simulink model "c02_SubAdc"  (R2024a)
settings: Solver=FixedStepDiscrete  StartTime=0.0  StopTime=1  FixedStep=mSim.dTime  MaxStep=Define.sModelSampleTime  RelTol=7.1420e-05
undefined symbols (not defined in the file): C02IGBTS, C02ITLKV, C02MTLKV, C02MTRTS, CnstNr
libraries: Lib_LPF x2
settings Model: Creator=user  LastModifiedBy=admin
settings SolverCC: MaxConsecutiveZCs=10000  ZeroCrossAlgorithm=Adaptive  AlgebraicLoopSolver=TrustRegion
settings DataIOCC: SaveOutput=off  DSMLogging=off  InspectSignalLogs=on  SaveTime=off  SignalLoggingName=logsout_Validator
settings OptimizationCC: BlockReduction=off  DefaultParameterBehavior=Inlined  UseDivisionForNetSlopeComputation=UseDivisionForReciprocalsOfIntegersOnly  GainParamInheritBuiltInType=on  UseFloatMulNetSlope=on  DefaultUnderspecifiedDataType=single  InlineInvariantSignals=on  BitwiseOrLogicalOp=Logical operator  PassReuseOutputArgsAs=Individual arguments  EfficientFloat2IntCast=on  LifeSpan=Inf  OptimizeBlockOrder=speed  DifferentSizesBufferReuse=on  EfficientTunableParamExpr=on
settings DebuggingCC: SignalInfNanChecking=error  SignalRangeChecking=error  ReadBeforeWriteMsg=EnableAllAsError  WriteAfterWriteMsg=EnableAllAsError  WriteAfterReadMsg=EnableAllAsError  AlgebraicLoopMsg=error  ArtificialAlgebraicLoopMsg=error  SaveWithDisabledLinksMsg=error  SaveWithParameterizedLinksMsg=error  BlockPriorityViolationMsg=error  SolverPrmCheckMsg=error  InheritedTsInSrcMsg=error  SingleTaskRateTransMsg=error  TasksWithSamePriorityMsg=error  SigSpecEnsureSampleTimeMsg=error  CheckMatrixSingularityMsg=error  IntegerOverflowMsg=error  ParameterUnderflowMsg=error  ParameterPrecisionLossMsg=error  ParameterTunabilityLossMsg=error  UnderSpecifiedDataTypeMsg=error  UnnecessaryDatatypeConvMsg=warning  VectorMatrixConversionMsg=error  SignalLabelMismatchMsg=error  UnconnectedInputMsg=error  UnconnectedOutputMsg=error  UnconnectedLineMsg=error  SFcnCompatibilityMsg=error  UniqueDataStoreMsg=error  BusObjectLabelMismatch=error  RootOutportRequireBusObject=error  AssertControl=DisableAll  ModelReferenceIOMismatchMessage=error  UnknownTsInhSupMsg=error  ModelReferenceDataLoggingMessage=error  ModelReferenceSymbolNameMessage=none  StateNameClashWarn=warning  StrictBusMsg=ErrorOnBusTreatedAsVector  NonBusSignalsTreatedAsBus=error  SFInvalidInputDataAccessInChartInitDiag=error  SFTransitionOutsideNaturalParentDiag=error  SFUnreachableExecutionPathDiag=error  SFUndirectedBroadcastEventsDiag=error  SFTransitionActionBeforeConditionDiag=error  SFTemporalDelaySmallerThanSampleTimeDiag=error  SFSelfTransitionDiag=error  SFExecutionAtInitializationDiag=error  IntegerSaturationMsg=error  UnitsInconsistencyMsg=none  VariantConditionMismatch=error
settings HardwareCC: ProdBitPerChar=16  ProdBitPerInt=16  ProdBitPerPointer=32  ProdBitPerSizeT=32  ProdBitPerPtrDiffT=32  ProdLargestAtomicInteger=Integer  ProdLargestAtomicFloat=None  ProdWordSize=16  ProdHWDeviceType=Texas Instruments->C2000
settings ModelReferenceCC: EnableRefExpFcnMdlSchedulingChecks=on  ModelReferenceNumInstancesAllowed=Single
settings SFSimCC: SimUseLocalCustomCode=off  CompileTimeRecursionLimit=0  EnableRuntimeRecursion=off  MATLABDynamicMemAlloc=off  CustomCodeUndefinedFunction=UseInterfaceOnly
settings RTWCC: Description=Embedded Coder  SystemTargetFile=ert.tlc  GenCodeOnly=on  TemplateMakefile=ert_default_tmf  GenerateReport=on  RTWUseLocalCustomCode=off  BuildConfiguration=Faster Runs  IncludeHyperlinkInReport=on  LaunchReport=on  GenerateTraceInfo=on  GenerateTraceReport=on  GenerateTraceReportSl=on  GenerateTraceReportSf=on  GenerateWebview=on  GenerateCodeMetricsReport=on  GenerateCodeReplacementReport=on  GPUComputeCapability=3.5  DLArmComputeVersion=19.05
settings CodeAppCC: ForceParamTrailComments=on  IgnoreCustomStorageClasses=off  MATLABFcnDesc=on  MangleLength=4  CustomSymbolStrGlobalVar=GvC02$N$M  CustomSymbolStrType=StrC02$N$M  CustomSymbolStrFcn=$N$M$F  CustomSymbolStrMacro=$N$M  DefineNamingRule=UpperCase  ParamNamingRule=UpperCase  SimulinkBlockComments=off  MATLABSourceComments=on  EnableCustomComments=on  ReqsInCode=on
settings ERTTargetCC: TargetLangStandard=C99 (ISO)  UtilityFuncGeneration=Shared location  MultiwordLength=2048  IncludeMdlTerminateFcn=off  CombineSignalStateStructs=on  SuppressErrorStatus=on  SupportAbsoluteTime=off  SupportNonFinite=off  ParenthesesLevel=Maximum  CastingMode=Standards  GenerateSharedConstants=off  InlinedParameterPlacement=NonHierarchical  ERTSrcFileBannerTemplate=t_code_template.cgt  ERTHdrFileBannerTemplate=t_code_template.cgt  ERTDataSrcFileTemplate=t_code_template.cgt  ERTDataHdrFileTemplate=t_code_template.cgt  ERTCustomFileTemplate=example_file_process.tlc  ERTFilePackagingFormat=CompactWithDataFile  PreserveExpressionOrder=on  SuppressUnreachableDefaultCases=off  EnableSignedLeftShifts=off  EnableSignedRightShifts=off  IndentStyle=Allman  IndentSize=4
settings ConfigComp: CovSaveName=coveragedata  CovMetricSettings=we  CovEnableCumulative=off  CovSaveCumulativeToWorkspaceVar=on  CovSaveSingleToWorkspaceVar=on  CovOutputDir=sldv_output/$ModelName$\sldv_covoutput  PSVerificationMode=BugFinder  PSModelRefIgnoreList=[]  PSEnableModelRefIgnoreList=off  PSModelRefMinMaxVerif=CheckAndConstrain  PSAutoStubLUT=on  DVModelCoverageObjectives=MCDC  DVTestSuiteOptimization=CombinedObjectives (Nonlinear Extended)  DVRebuildModelRepresentation=Always
settings SimscapeCC: SimscapeNormalizeSystem=off

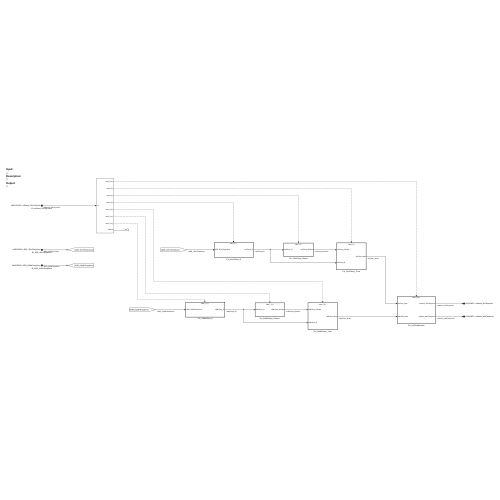
[thumbnail: Simulink's stored preview of the top-level diagram]
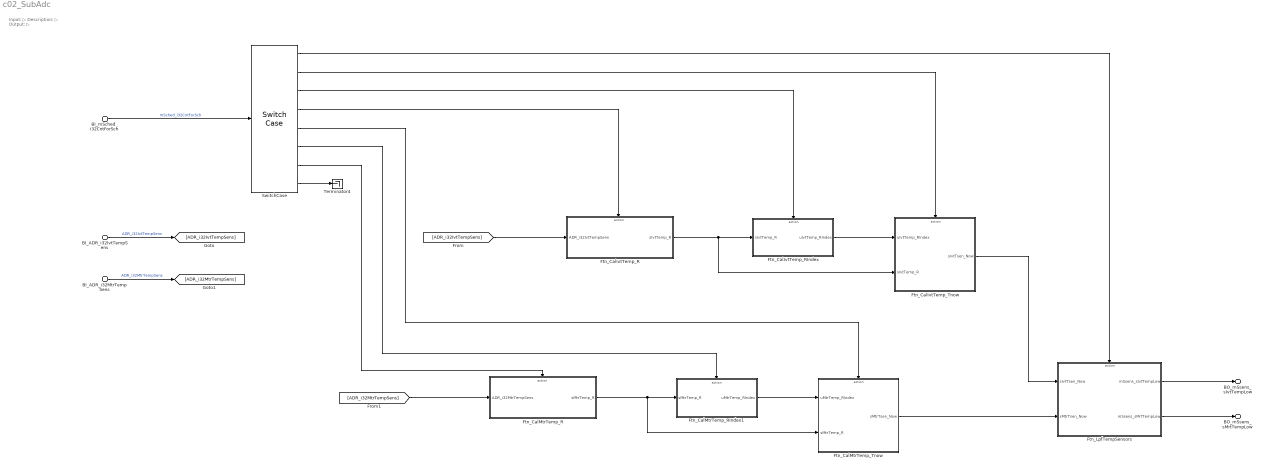
== system c02_SubAdc ==
  note: Input:
      | ▷
      | Description:
      | ▷
      | Output:
      | ▷
  BI_ADR_i32IvtTempSens : Inport  Description=■ 설명: IGBT 온도 센서 ADCV  PortName=bADCREAD  Element=ADR_i32IvtTempSens
  BI_ADR_i32MtrTempSens : Inport  Description=■ 설명: 모터 온도 센서 ADCV  PortName=bADCREAD  Element=ADR_i32MtrTempSens
  BI_mSched_i32CntForSch : Inport  Description=■ 설명: 메인 스케쥴 카운터  Port=2  PortName=bB01SCHED  Element=mSched_i32CntForSch
  Ftn_CalIvtTemp_R : Subsystem
      settings: RTWSystemCode=Nonreusable function  RTWFcnNameOpts=Use subsystem name
  Ftn_CalIvtTemp_RIndex : Subsystem
      settings: RTWSystemCode=Nonreusable function  RTWFcnNameOpts=Use subsystem name
  Ftn_CalIvtTemp_Tnow : Subsystem
      settings: RTWSystemCode=Nonreusable function  RTWFcnNameOpts=Use subsystem name
  Ftn_CalMtrTemp_R : Subsystem
      settings: RTWSystemCode=Nonreusable function  RTWFcnNameOpts=Use subsystem name
  Ftn_CalMtrTemp_RIndex1 : Subsystem
      settings: RTWSystemCode=Nonreusable function  RTWFcnNameOpts=Use subsystem name
  Ftn_CalMtrTemp_Tnow : Subsystem
      settings: RTWSystemCode=Nonreusable function  RTWFcnNameOpts=Use subsystem name
  Ftn_LpfTempSensors : Subsystem
  SwitchCase : SwitchCase  CaseConditions={22, 6,4,2,16,14,12}
  Terminator4 : Terminator
  BO_mSsens_sIvtTempLow : Outport  Description=■ 설명: IGBT 온도  PortName=bC02SADC  Element=mSsens_sIvtTempLow
  BO_mSsens_sMrtTempLow : Outport  Description=■ 설명: 모터 온도  PortName=bC02SADC  Element=mSsens_sMrtTempLow
  wires:
  BI_ADR_i32IvtTempSens/1 -> [ADR_i32IvtTempSens]  "ADR_i32IvtTempSens"
  BI_mSched_i32CntForSch/1 -> SwitchCase/1  "mSched_i32CntForSch"
  Ftn_CalIvtTemp_R/1(sIvtTemp_R) -> Ftn_CalIvtTemp_RIndex/1(sIvtTemp_R), Ftn_CalIvtTemp_Tnow/2(sIvtTemp_R)
  Ftn_CalIvtTemp_RIndex/1(uIvtTemp_RIndex) -> Ftn_CalIvtTemp_Tnow/1(uIvtTemp_RIndex)
  SwitchCase/2 -> Ftn_CalIvtTemp_Tnow/Action
  SwitchCase/3 -> Ftn_CalIvtTemp_RIndex/Action
  SwitchCase/4 -> Ftn_CalIvtTemp_R/Action
  [ADR_i32IvtTempSens] -> Ftn_CalIvtTemp_R/1(ADR_i32IvtTempSens)
  Ftn_CalIvtTemp_Tnow/1(sIvtTsen_Now) -> Ftn_LpfTempSensors/1(sIvtTsen_Now)
  BI_ADR_i32MtrTempSens/1 -> [ADR_i32MtrTempSens]  "ADR_i32MtrTempSens"
  SwitchCase/8 -> Terminator4/1
  SwitchCase/1 -> Ftn_LpfTempSensors/Action
  Ftn_LpfTempSensors/1(mSsens_sIvtTempLow) -> BO_mSsens_sIvtTempLow/1
  Ftn_LpfTempSensors/2(mSsens_sMrtTempLow) -> BO_mSsens_sMrtTempLow/1
  Ftn_CalMtrTemp_Tnow/1(sMtrTsen_Now) -> Ftn_LpfTempSensors/2(sMtrTsen_Now)
  Ftn_CalMtrTemp_RIndex1/1(uMtrTemp_RIndex) -> Ftn_CalMtrTemp_Tnow/1(uMtrTemp_RIndex)
  Ftn_CalMtrTemp_R/1(sMtrTemp_R) -> Ftn_CalMtrTemp_RIndex1/1(sMtrTemp_R), Ftn_CalMtrTemp_Tnow/2(sMtrTemp_R)
  [ADR_i32MtrTempSens] -> Ftn_CalMtrTemp_R/1(ADR_i32MtrTempSens)
  SwitchCase/7 -> Ftn_CalMtrTemp_R/Action
  SwitchCase/6 -> Ftn_CalMtrTemp_RIndex1/Action
  SwitchCase/5 -> Ftn_CalMtrTemp_Tnow/Action

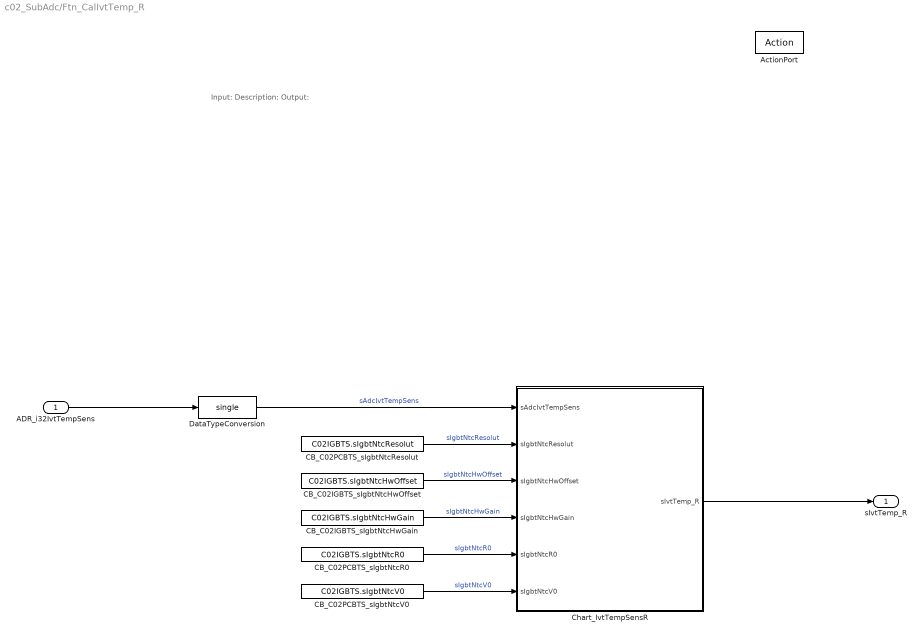
== system c02_SubAdc/Ftn_CalIvtTemp_R ==
  note: Input:
      | Description:
      | Output:
  ADR_i32IvtTempSens : Inport  OutMin=0  OutMax=4095
  ActionPort : ActionPort  ActionPortLabel=case [ 2 ]:
  CB_C02IGBTS_sIgbtNtcHwGain : Constant  Value=C02IGBTS.sIgbtNtcHwGain
  CB_C02IGBTS_sIgbtNtcHwOffset : Constant  Value=C02IGBTS.sIgbtNtcHwOffset
  CB_C02PCBTS_sIgbtNtcR0 : Constant  Value=C02IGBTS.sIgbtNtcR0
  CB_C02PCBTS_sIgbtNtcResolut : Constant  Value=C02IGBTS.sIgbtNtcResolut
  CB_C02PCBTS_sIgbtNtcV0 : Constant  Value=C02IGBTS.sIgbtNtcV0
  Chart_IvtTempSensR : Stateflow chart  TreatAsAtomicUnit=on  RTWFileName=Sensor
      settings: RTWFcnNameOpts=Use subsystem name  RTWFileNameOpts=User specified
  DataTypeConversion : DataTypeConversion  OutDataTypeStr=single  SaturateOnIntegerOverflow=off  RndMeth=Floor
  sIvtTemp_R : Outport  OutMin=0  OutMax=4.9e+05
  wires:
  Chart_IvtTempSensR/1(sIvtTemp_R) -> sIvtTemp_R/1
  ADR_i32IvtTempSens/1 -> DataTypeConversion/1
  CB_C02PCBTS_sIgbtNtcV0/1 -> Chart_IvtTempSensR/6(sIgbtNtcV0)  "sIgbtNtcV0"
  CB_C02PCBTS_sIgbtNtcResolut/1 -> Chart_IvtTempSensR/2(sIgbtNtcResolut)  "sIgbtNtcResolut"
  CB_C02PCBTS_sIgbtNtcR0/1 -> Chart_IvtTempSensR/5(sIgbtNtcR0)  "sIgbtNtcR0"
  DataTypeConversion/1 -> Chart_IvtTempSensR/1(sAdcIvtTempSens)  "sAdcIvtTempSens"
  CB_C02IGBTS_sIgbtNtcHwOffset/1 -> Chart_IvtTempSensR/3(sIgbtNtcHwOffset)  "sIgbtNtcHwOffset"
  CB_C02IGBTS_sIgbtNtcHwGain/1 -> Chart_IvtTempSensR/4(sIgbtNtcHwGain)  "sIgbtNtcHwGain"

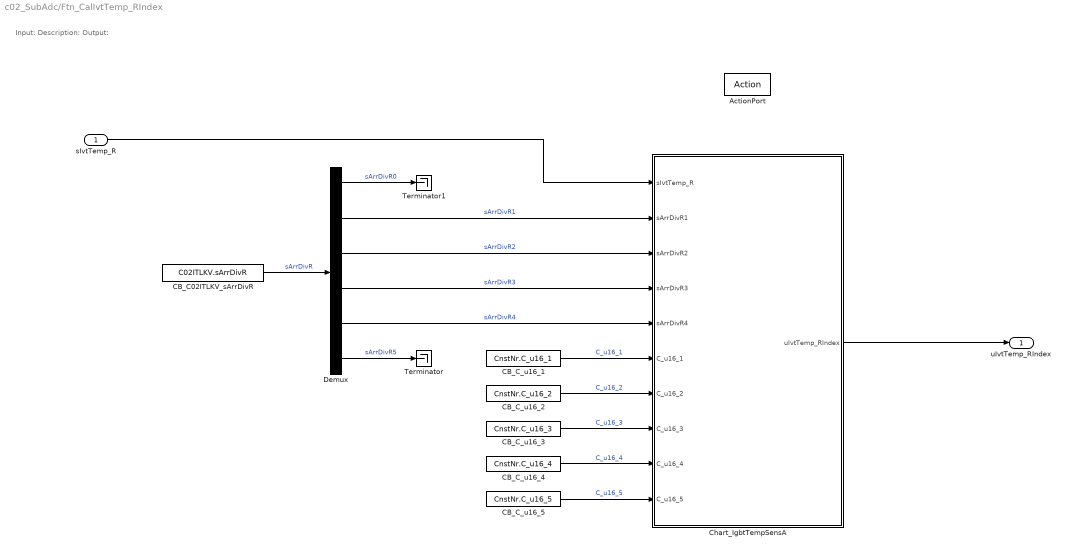
== system c02_SubAdc/Ftn_CalIvtTemp_RIndex ==
  note: Input:
      | Description:
      | Output:
  sIvtTemp_R : Inport  OutMin=0  OutMax=4.9e+05
  ActionPort : ActionPort  ActionPortLabel=case [ 4 ]:
  CB_C02ITLKV_sArrDivR : Constant  Value=C02ITLKV.sArrDivR  OutDataTypeStr=single
  CB_C_u16_1 : Constant  Value=CnstNr.C_u16_1
  CB_C_u16_2 : Constant  Value=CnstNr.C_u16_2
  CB_C_u16_3 : Constant  Value=CnstNr.C_u16_3
  CB_C_u16_4 : Constant  Value=CnstNr.C_u16_4
  CB_C_u16_5 : Constant  Value=CnstNr.C_u16_5
  Chart_IgbtTempSensA : Stateflow chart  TreatAsAtomicUnit=on
  Demux : Demux  Outputs=6
  Terminator : Terminator
  Terminator1 : Terminator
  uIvtTemp_RIndex : Outport  OutMin=1  OutMax=5  VectorParamsAs1DForOutWhenUnconnected=off
  wires:
  Chart_IgbtTempSensA/1(uIvtTemp_RIndex) -> uIvtTemp_RIndex/1
  sIvtTemp_R/1 -> Chart_IgbtTempSensA/1(sIvtTemp_R)
  CB_C_u16_3/1 -> Chart_IgbtTempSensA/8(C_u16_3)  "C_u16_3"
  CB_C_u16_1/1 -> Chart_IgbtTempSensA/6(C_u16_1)  "C_u16_1"
  CB_C_u16_4/1 -> Chart_IgbtTempSensA/9(C_u16_4)  "C_u16_4"
  CB_C_u16_5/1 -> Chart_IgbtTempSensA/10(C_u16_5)  "C_u16_5"
  CB_C_u16_2/1 -> Chart_IgbtTempSensA/7(C_u16_2)  "C_u16_2"
  CB_C02ITLKV_sArrDivR/1 -> Demux/1  "sArrDivR"
  Demux/3 -> Chart_IgbtTempSensA/3(sArrDivR2)  "sArrDivR2"
  Demux/5 -> Chart_IgbtTempSensA/5(sArrDivR4)  "sArrDivR4"
  Demux/4 -> Chart_IgbtTempSensA/4(sArrDivR3)  "sArrDivR3"
  Demux/1 -> Terminator1/1  "sArrDivR0"
  Demux/2 -> Chart_IgbtTempSensA/2(sArrDivR1)  "sArrDivR1"
  Demux/6 -> Terminator/1  "sArrDivR5"

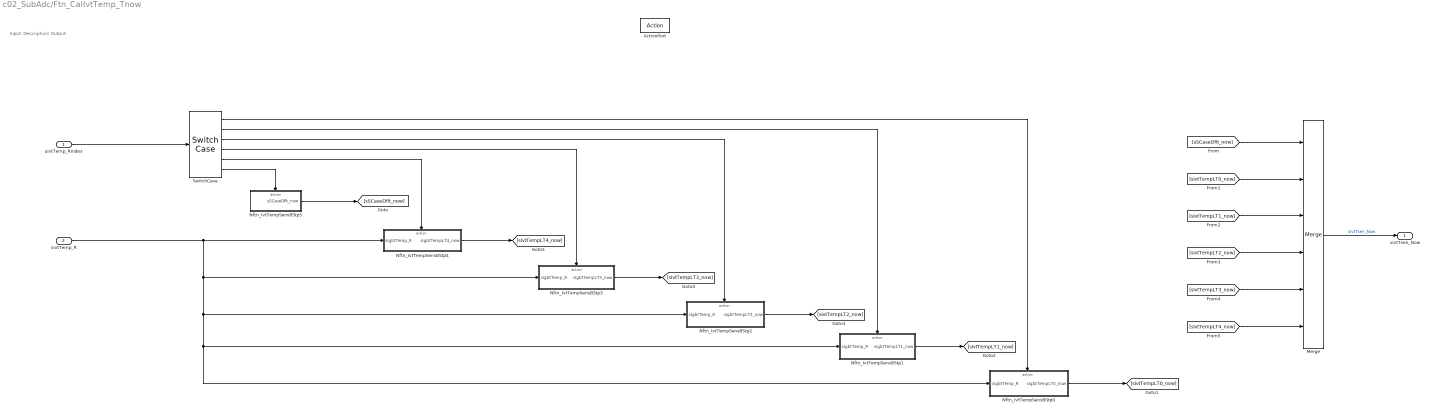
== system c02_SubAdc/Ftn_CalIvtTemp_Tnow ==
  note: Input:
      | Description:
      | Output:
  uIvtTemp_RIndex : Inport  OutMin=1  OutMax=5
  sIvtTemp_R : Inport  Port=2  OutMin=0  OutMax=4.9e+05
  ActionPort : ActionPort  ActionPortLabel=case [ 6 ]:
  Merge : Merge  Inputs=6
  Nftn_IvtTempSensBStp0 : Subsystem
      settings: RTWSystemCode=Inline  RTWFcnNameOpts=Use subsystem name
  Nftn_IvtTempSensBStp1 : Subsystem
      settings: RTWSystemCode=Inline  RTWFcnNameOpts=Use subsystem name
  Nftn_IvtTempSensBStp2 : Subsystem
      settings: RTWSystemCode=Inline  RTWFcnNameOpts=Use subsystem name
  Nftn_IvtTempSensBStp3 : Subsystem
      settings: RTWSystemCode=Inline  RTWFcnNameOpts=Use subsystem name
  Nftn_IvtTempSensBStp4 : Subsystem
      settings: RTWSystemCode=Inline  RTWFcnNameOpts=Use subsystem name
  Nftn_IvtTempSensBStp5 : Subsystem
      settings: RTWSystemCode=Inline  RTWFcnNameOpts=Use subsystem name
  SwitchCase : SwitchCase  CaseConditions={1,2,3,4,5}
  sIvtTsen_Now : Outport  OutMin=-6.918  OutMax=233.8805  VectorParamsAs1DForOutWhenUnconnected=off
  wires:
  Nftn_IvtTempSensBStp4/1(sIgbtTempLT4_now) -> [sIvtTempLT4_now]
  SwitchCase/1 -> Nftn_IvtTempSensBStp0/Action
  SwitchCase/2 -> Nftn_IvtTempSensBStp1/Action
  SwitchCase/3 -> Nftn_IvtTempSensBStp2/Action
  SwitchCase/4 -> Nftn_IvtTempSensBStp3/Action
  SwitchCase/5 -> Nftn_IvtTempSensBStp4/Action
  Nftn_IvtTempSensBStp3/1(sIgbtTempLT3_now) -> [sIvtTempLT3_now]
  Nftn_IvtTempSensBStp2/1(sIgbtTempLT2_now) -> [sIvtTempLT2_now]
  Nftn_IvtTempSensBStp1/1(sIgbtTempLT1_now) -> [sIvtTempLT1_now]
  Nftn_IvtTempSensBStp0/1(sIgbtTempLT0_now) -> [sIvtTempLT0_now]
  Nftn_IvtTempSensBStp5/1(sSCaseDflt_now) -> [sSCaseDflt_now]
  [sIvtTempLT4_now] -> Merge/6
  [sIvtTempLT3_now] -> Merge/5
  [sIvtTempLT2_now] -> Merge/4
  [sIvtTempLT1_now] -> Merge/3
  [sIvtTempLT0_now] -> Merge/2
  [sSCaseDflt_now] -> Merge/1
  SwitchCase/6 -> Nftn_IvtTempSensBStp5/Action
  sIvtTemp_R/1 -> Nftn_IvtTempSensBStp0/1(sIgbtTemp_R), Nftn_IvtTempSensBStp1/1(sIgbtTemp_R), Nftn_IvtTempSensBStp2/1(sIgbtTemp_R), Nftn_IvtTempSensBStp3/1(sIgbtTemp_R), Nftn_IvtTempSensBStp4/1(sIgbtTemp_R)
  Merge/1 -> sIvtTsen_Now/1  "sIvtTsen_Now"
  uIvtTemp_RIndex/1 -> SwitchCase/1

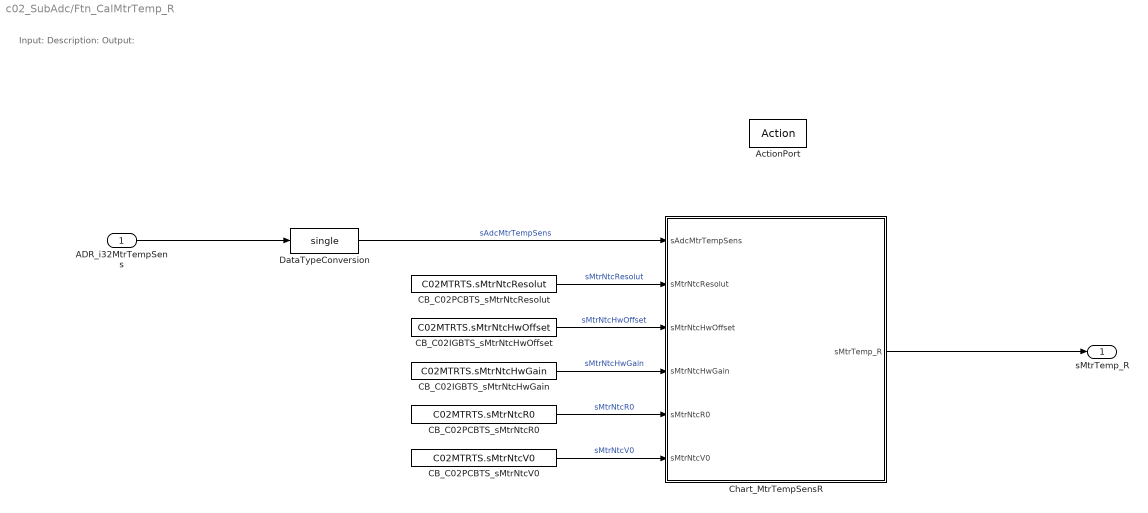
== system c02_SubAdc/Ftn_CalMtrTemp_R ==
  note: Input:
      | Description:
      | Output:
  ADR_i32MtrTempSens : Inport  OutMin=0  OutMax=4095
  ActionPort : ActionPort  ActionPortLabel=case [ 12 ]:
  CB_C02IGBTS_sMtrNtcHwGain : Constant  Value=C02MTRTS.sMtrNtcHwGain
  CB_C02IGBTS_sMtrNtcHwOffset : Constant  Value=C02MTRTS.sMtrNtcHwOffset
  CB_C02PCBTS_sMtrNtcR0 : Constant  Value=C02MTRTS.sMtrNtcR0
  CB_C02PCBTS_sMtrNtcResolut : Constant  Value=C02MTRTS.sMtrNtcResolut
  CB_C02PCBTS_sMtrNtcV0 : Constant  Value=C02MTRTS.sMtrNtcV0
  Chart_MtrTempSensR : Stateflow chart  TreatAsAtomicUnit=on  RTWFileName=Sensor
      settings: RTWFcnNameOpts=Use subsystem name  RTWFileNameOpts=User specified
  DataTypeConversion : DataTypeConversion  OutDataTypeStr=single  SaturateOnIntegerOverflow=off  RndMeth=Floor
  sMtrTemp_R : Outport  OutMin=0  OutMax=4.9e+05
  wires:
  CB_C02IGBTS_sMtrNtcHwGain/1 -> Chart_MtrTempSensR/4(sMtrNtcHwGain)  "sMtrNtcHwGain"
  CB_C02IGBTS_sMtrNtcHwOffset/1 -> Chart_MtrTempSensR/3(sMtrNtcHwOffset)  "sMtrNtcHwOffset"
  DataTypeConversion/1 -> Chart_MtrTempSensR/1(sAdcMtrTempSens)  "sAdcMtrTempSens"
  CB_C02PCBTS_sMtrNtcR0/1 -> Chart_MtrTempSensR/5(sMtrNtcR0)  "sMtrNtcR0"
  CB_C02PCBTS_sMtrNtcResolut/1 -> Chart_MtrTempSensR/2(sMtrNtcResolut)  "sMtrNtcResolut"
  CB_C02PCBTS_sMtrNtcV0/1 -> Chart_MtrTempSensR/6(sMtrNtcV0)  "sMtrNtcV0"
  ADR_i32MtrTempSens/1 -> DataTypeConversion/1
  Chart_MtrTempSensR/1(sMtrTemp_R) -> sMtrTemp_R/1

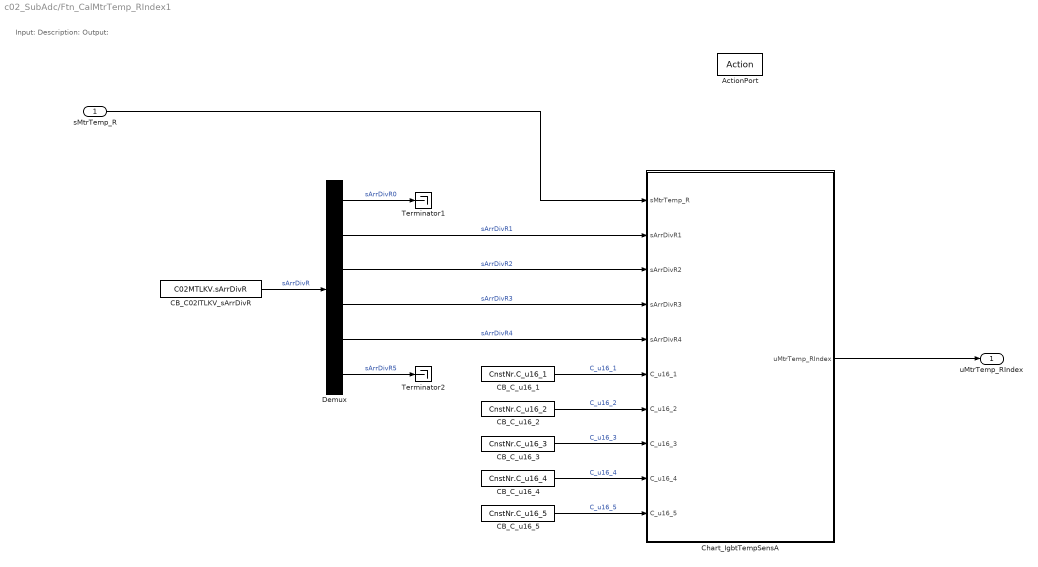
== system c02_SubAdc/Ftn_CalMtrTemp_RIndex1 ==
  note: Input:
      | Description:
      | Output:
  sMtrTemp_R : Inport  OutMin=0  OutMax=4.9e+05
  ActionPort : ActionPort  ActionPortLabel=case [ 14 ]:
  CB_C02ITLKV_sArrDivR : Constant  Value=C02MTLKV.sArrDivR  OutDataTypeStr=single
  CB_C_u16_1 : Constant  Value=CnstNr.C_u16_1
  CB_C_u16_2 : Constant  Value=CnstNr.C_u16_2
  CB_C_u16_3 : Constant  Value=CnstNr.C_u16_3
  CB_C_u16_4 : Constant  Value=CnstNr.C_u16_4
  CB_C_u16_5 : Constant  Value=CnstNr.C_u16_5
  Chart_IgbtTempSensA : Stateflow chart  TreatAsAtomicUnit=on
  Demux : Demux  Outputs=6
  Terminator1 : Terminator
  Terminator2 : Terminator
  uMtrTemp_RIndex : Outport  OutMin=1  OutMax=5  VectorParamsAs1DForOutWhenUnconnected=off
  wires:
  Demux/1 -> Terminator1/1  "sArrDivR0"
  CB_C02ITLKV_sArrDivR/1 -> Demux/1  "sArrDivR"
  CB_C_u16_2/1 -> Chart_IgbtTempSensA/7(C_u16_2)  "C_u16_2"
  CB_C_u16_5/1 -> Chart_IgbtTempSensA/10(C_u16_5)  "C_u16_5"
  CB_C_u16_4/1 -> Chart_IgbtTempSensA/9(C_u16_4)  "C_u16_4"
  CB_C_u16_1/1 -> Chart_IgbtTempSensA/6(C_u16_1)  "C_u16_1"
  CB_C_u16_3/1 -> Chart_IgbtTempSensA/8(C_u16_3)  "C_u16_3"
  sMtrTemp_R/1 -> Chart_IgbtTempSensA/1(sMtrTemp_R)
  Chart_IgbtTempSensA/1(uMtrTemp_RIndex) -> uMtrTemp_RIndex/1
  Demux/2 -> Chart_IgbtTempSensA/2(sArrDivR1)  "sArrDivR1"
  Demux/3 -> Chart_IgbtTempSensA/3(sArrDivR2)  "sArrDivR2"
  Demux/4 -> Chart_IgbtTempSensA/4(sArrDivR3)  "sArrDivR3"
  Demux/5 -> Chart_IgbtTempSensA/5(sArrDivR4)  "sArrDivR4"
  Demux/6 -> Terminator2/1  "sArrDivR5"

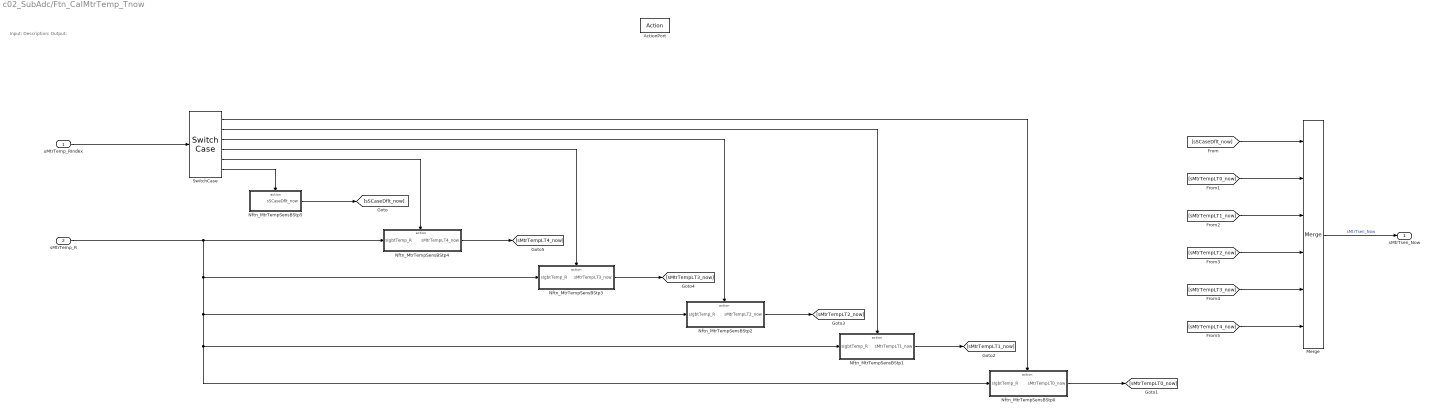
== system c02_SubAdc/Ftn_CalMtrTemp_Tnow ==
  note: Input:
      | Description:
      | Output:
  uMtrTemp_RIndex : Inport  OutMin=1  OutMax=5
  sMtrTemp_R : Inport  Port=2  OutMin=0  OutMax=4.9e+05
  ActionPort : ActionPort  ActionPortLabel=case [ 16 ]:
  Merge : Merge  Inputs=6
  Nftn_MtrTempSensBStp0 : Subsystem
      settings: RTWSystemCode=Inline  RTWFcnNameOpts=Use subsystem name
  Nftn_MtrTempSensBStp1 : Subsystem
      settings: RTWSystemCode=Inline  RTWFcnNameOpts=Use subsystem name
  Nftn_MtrTempSensBStp2 : Subsystem
      settings: RTWSystemCode=Inline  RTWFcnNameOpts=Use subsystem name
  Nftn_MtrTempSensBStp3 : Subsystem
      settings: RTWSystemCode=Inline  RTWFcnNameOpts=Use subsystem name
  Nftn_MtrTempSensBStp4 : Subsystem
      settings: RTWSystemCode=Inline  RTWFcnNameOpts=Use subsystem name
  Nftn_MtrTempSensBStp5 : Subsystem
      settings: RTWSystemCode=Inline  RTWFcnNameOpts=Use subsystem name
  SwitchCase : SwitchCase  CaseConditions={1,2,3,4,5}
  sMtrTsen_Now : Outport  OutMin=-6.918  OutMax=233.8805  VectorParamsAs1DForOutWhenUnconnected=off
  wires:
  uMtrTemp_RIndex/1 -> SwitchCase/1
  Merge/1 -> sMtrTsen_Now/1  "sMtrTsen_Now"
  sMtrTemp_R/1 -> Nftn_MtrTempSensBStp4/1(sIgbtTemp_R), Nftn_MtrTempSensBStp3/1(sIgbtTemp_R), Nftn_MtrTempSensBStp2/1(sIgbtTemp_R), Nftn_MtrTempSensBStp1/1(sIgbtTemp_R), Nftn_MtrTempSensBStp0/1(sIgbtTemp_R)
  SwitchCase/6 -> Nftn_MtrTempSensBStp5/Action
  [sSCaseDflt_now] -> Merge/1
  [sMtrTempLT0_now] -> Merge/2
  [sMtrTempLT1_now] -> Merge/3
  [sMtrTempLT2_now] -> Merge/4
  [sMtrTempLT3_now] -> Merge/5
  [sMtrTempLT4_now] -> Merge/6
  Nftn_MtrTempSensBStp5/1(sSCaseDflt_now) -> [sSCaseDflt_now]
  Nftn_MtrTempSensBStp0/1(sMtrTempLT0_now) -> [sMtrTempLT0_now]
  Nftn_MtrTempSensBStp1/1(sMtrTempLT1_now) -> [sMtrTempLT1_now]
  Nftn_MtrTempSensBStp2/1(sMtrTempLT2_now) -> [sMtrTempLT2_now]
  Nftn_MtrTempSensBStp3/1(sMtrTempLT3_now) -> [sMtrTempLT3_now]
  SwitchCase/5 -> Nftn_MtrTempSensBStp4/Action
  SwitchCase/4 -> Nftn_MtrTempSensBStp3/Action
  SwitchCase/3 -> Nftn_MtrTempSensBStp2/Action
  SwitchCase/2 -> Nftn_MtrTempSensBStp1/Action
  SwitchCase/1 -> Nftn_MtrTempSensBStp0/Action
  Nftn_MtrTempSensBStp4/1(sMtrTempLT4_now) -> [sMtrTempLT4_now]

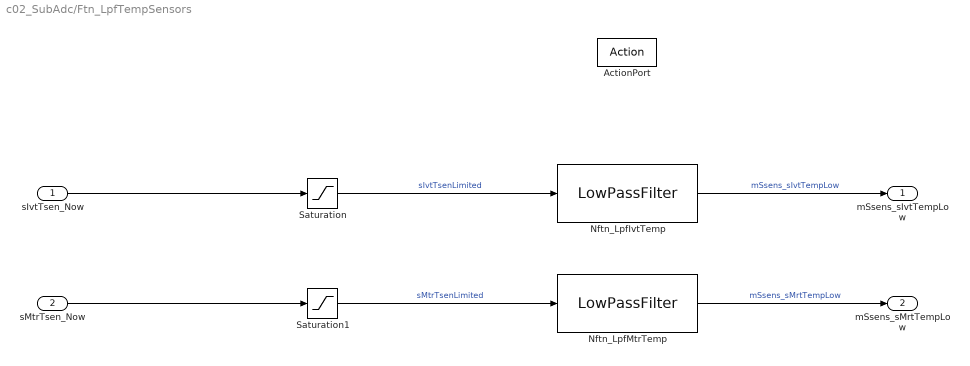
== system c02_SubAdc/Ftn_LpfTempSensors ==
  sIvtTsen_Now : Inport
  sMtrTsen_Now : Inport  Port=2
  ActionPort : ActionPort  ActionPortLabel=case [ 22 ]:
  Nftn_LpfIvtTemp : Lib_LPF/LowPassFilter  La=C02IGBTS.sTempLa  Lb=C02IGBTS.sTempLb  Init_Value=C02IGBTS.sTempInit
  Nftn_LpfMtrTemp : Lib_LPF/LowPassFilter  La=C02MTRTS.sTempLa  Lb=C02MTRTS.sTempLb  Init_Value=C02MTRTS.sTempInit
  Saturation : Saturate  UpperLimit=C02IGBTS.sIgbtNtcTmax  LowerLimit=C02IGBTS.sIgbtNtcTmin
  Saturation1 : Saturate  UpperLimit=C02MTRTS.sMtrNtcTmax  LowerLimit=C02MTRTS.sMtrNtcTmin
  mSsens_sIvtTempLow : Outport
  mSsens_sMrtTempLow : Outport  Port=2
  wires:
  Nftn_LpfIvtTemp/1 -> mSsens_sIvtTempLow/1  "mSsens_sIvtTempLow"
  sIvtTsen_Now/1 -> Saturation/1
  Nftn_LpfMtrTemp/1 -> mSsens_sMrtTempLow/1  "mSsens_sMrtTempLow"
  Saturation1/1 -> Nftn_LpfMtrTemp/1  "sMtrTsenLimited"
  Saturation/1 -> Nftn_LpfIvtTemp/1  "sIvtTsenLimited"
  sMtrTsen_Now/1 -> Saturation1/1

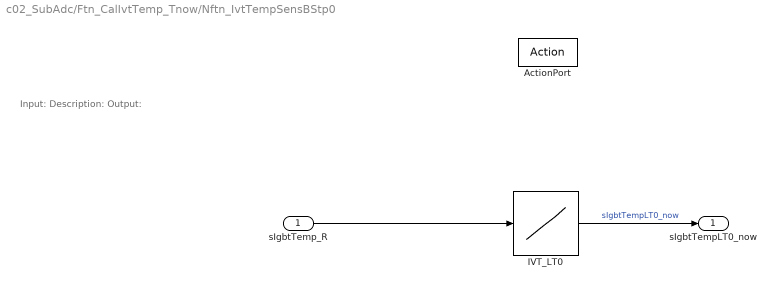
== system c02_SubAdc/Ftn_CalIvtTemp_Tnow/Nftn_IvtTempSensBStp0 ==
  note: Input:
      | Description:
      | Output:
  sIgbtTemp_R : Inport  Description=|  OutMin=0  OutMax=4.9e+05
      | ■ 대표값: 2062
      | ■ 설명: Igbt 온도 센서의 저항값
      settings: AttributesFormatString=|
      | ■ SWC Name: %<Parent>
      | ■ DataType: single
      | ■ Max: %<OutMax>
      | ■ Min: %<OutMin>
      | %<Description>
  ActionPort : ActionPort  ActionPortLabel=case [ 1 ]:
  IVT_LT0 : Lookup_n-D  NumberOfTableDimensions=1  BreakpointsForDimension1=C02ITLKV.sArrR0  Table=C02ITLKV.sArrT0  ExtrapMethod=Clip  UseLastTableValue=on  InternalRulePriority=Speed
      settings: AttributesFormatString=%<UseLastTableValue>
  sIgbtTempLT0_now : Outport
  wires:
  IVT_LT0/1 -> sIgbtTempLT0_now/1  "sIgbtTempLT0_now"
  sIgbtTemp_R/1 -> IVT_LT0/1

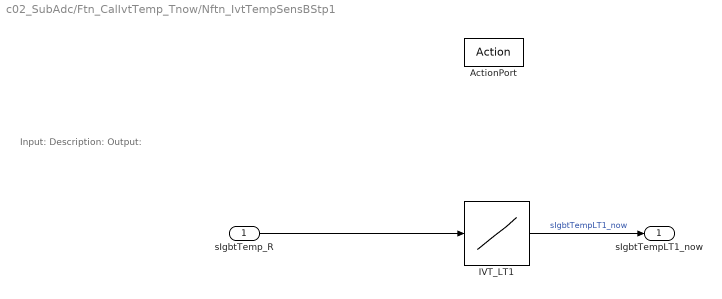
== system c02_SubAdc/Ftn_CalIvtTemp_Tnow/Nftn_IvtTempSensBStp1 ==
  note: Input:
      | Description:
      | Output:
  sIgbtTemp_R : Inport  Description=|  OutMin=0  OutMax=4.9e+05
      | ■ 대표값: 2062
      | ■ 설명: Igbt 온도 센서의 저항값
      settings: AttributesFormatString=|
      | ■ SWC Name: %<Parent>
      | ■ DataType: single
      | ■ Max: %<OutMax>
      | ■ Min: %<OutMin>
      | %<Description>
  ActionPort : ActionPort  ActionPortLabel=case [ 2 ]:
  IVT_LT1 : Lookup_n-D  NumberOfTableDimensions=1  BreakpointsForDimension1=C02ITLKV.sArrR1  Table=C02ITLKV.sArrT1  ExtrapMethod=Clip  UseLastTableValue=on  InternalRulePriority=Speed
      settings: AttributesFormatString=%<UseLastTableValue>
  sIgbtTempLT1_now : Outport
  wires:
  sIgbtTemp_R/1 -> IVT_LT1/1
  IVT_LT1/1 -> sIgbtTempLT1_now/1  "sIgbtTempLT1_now"

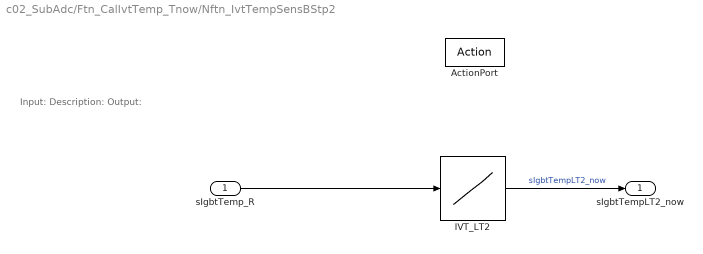
== system c02_SubAdc/Ftn_CalIvtTemp_Tnow/Nftn_IvtTempSensBStp2 ==
  note: Input:
      | Description:
      | Output:
  sIgbtTemp_R : Inport  Description=|  OutMin=0  OutMax=4.9e+05
      | ■ 대표값: 2062
      | ■ 설명: Igbt 온도 센서의 저항값
      settings: AttributesFormatString=|
      | ■ SWC Name: %<Parent>
      | ■ DataType: single
      | ■ Max: %<OutMax>
      | ■ Min: %<OutMin>
      | %<Description>
  ActionPort : ActionPort  ActionPortLabel=case [ 3 ]:
  IVT_LT2 : Lookup_n-D  NumberOfTableDimensions=1  BreakpointsForDimension1=C02ITLKV.sArrR2  Table=C02ITLKV.sArrT2  ExtrapMethod=Clip  UseLastTableValue=on  InternalRulePriority=Speed
      settings: AttributesFormatString=%<UseLastTableValue>
  sIgbtTempLT2_now : Outport
  wires:
  IVT_LT2/1 -> sIgbtTempLT2_now/1  "sIgbtTempLT2_now"
  sIgbtTemp_R/1 -> IVT_LT2/1

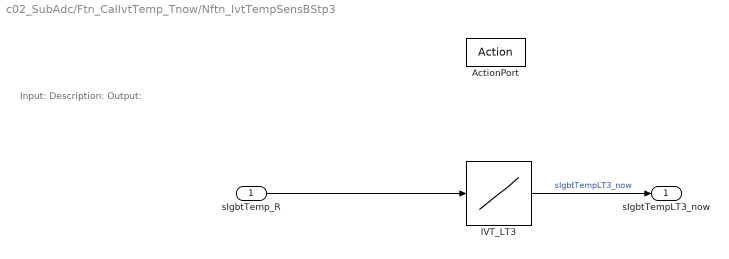
== system c02_SubAdc/Ftn_CalIvtTemp_Tnow/Nftn_IvtTempSensBStp3 ==
  note: Input:
      | Description:
      | Output:
  sIgbtTemp_R : Inport  Description=|  OutMin=0  OutMax=4.9e+05
      | ■ 대표값: 2062
      | ■ 설명: Igbt 온도 센서의 저항값
      settings: AttributesFormatString=|
      | ■ SWC Name: %<Parent>
      | ■ DataType: single
      | ■ Max: %<OutMax>
      | ■ Min: %<OutMin>
      | %<Description>
  ActionPort : ActionPort  ActionPortLabel=case [ 4 ]:
  IVT_LT3 : Lookup_n-D  NumberOfTableDimensions=1  BreakpointsForDimension1=C02ITLKV.sArrR3  Table=C02ITLKV.sArrT3  ExtrapMethod=Clip  UseLastTableValue=on  InternalRulePriority=Speed
      settings: AttributesFormatString=%<UseLastTableValue>
  sIgbtTempLT3_now : Outport
  wires:
  sIgbtTemp_R/1 -> IVT_LT3/1
  IVT_LT3/1 -> sIgbtTempLT3_now/1  "sIgbtTempLT3_now"

== system c02_SubAdc/Ftn_CalIvtTemp_Tnow/Nftn_IvtTempSensBStp4 ==
  note: Input:
      | Description:
      | Output:
  sIgbtTemp_R : Inport  Description=|  OutMin=0  OutMax=4.9e+05
      | ■ 대표값: 2062
      | ■ 설명: Igbt 온도 센서의 저항값
  ActionPort : ActionPort  ActionPortLabel=case [ 5 ]:
  IVT_LT4 : Lookup_n-D  NumberOfTableDimensions=1  BreakpointsForDimension1=C02ITLKV.sArrR4  Table=C02ITLKV.sArrT4  ExtrapMethod=Clip  UseLastTableValue=on  InternalRulePriority=Speed
      settings: AttributesFormatString=%<UseLastTableValue>
  sIgbtTempLT4_now : Outport
  wires:
  IVT_LT4/1 -> sIgbtTempLT4_now/1  "sIgbtTempLT4_now"
  sIgbtTemp_R/1 -> IVT_LT4/1

== system c02_SubAdc/Ftn_CalIvtTemp_Tnow/Nftn_IvtTempSensBStp5 ==
  note: Input:
      | Description:
      | Output:
  ActionPort : ActionPort  ActionPortLabel=default:
  CB_sSCaseDflt_now : Constant  Value=0  OutDataTypeStr=single
  sSCaseDflt_now : Outport
  wires:
  CB_sSCaseDflt_now/1 -> sSCaseDflt_now/1  "sSCaseDflt_now"

== system c02_SubAdc/Ftn_CalMtrTemp_Tnow/Nftn_MtrTempSensBStp0 ==
  note: Input:
      | Description:
      | Output:
  sIgbtTemp_R : Inport  Description=|  OutMin=0  OutMax=4.9e+05
      | ■ 대표값: 2062
      | ■ 설명: Igbt 온도 센서의 저항값
      settings: AttributesFormatString=|
      | ■ SWC Name: %<Parent>
      | ■ DataType: single
      | ■ Max: %<OutMax>
      | ■ Min: %<OutMin>
      | %<Description>
  ActionPort : ActionPort  ActionPortLabel=case [ 1 ]:
  IVT_LT0 : Lookup_n-D  NumberOfTableDimensions=1  BreakpointsForDimension1=C02MTLKV.sArrR0  Table=C02MTLKV.sArrT0  ExtrapMethod=Clip  UseLastTableValue=on  InternalRulePriority=Speed
      settings: AttributesFormatString=%<UseLastTableValue>
  sMtrTempLT0_now : Outport
  wires:
  sIgbtTemp_R/1 -> IVT_LT0/1
  IVT_LT0/1 -> sMtrTempLT0_now/1  "sMtrTempLT0_now"

== system c02_SubAdc/Ftn_CalMtrTemp_Tnow/Nftn_MtrTempSensBStp1 ==
  note: Input:
      | Description:
      | Output:
  sIgbtTemp_R : Inport  Description=|  OutMin=0  OutMax=4.9e+05
      | ■ 대표값: 2062
      | ■ 설명: Igbt 온도 센서의 저항값
      settings: AttributesFormatString=|
      | ■ SWC Name: %<Parent>
      | ■ DataType: single
      | ■ Max: %<OutMax>
      | ■ Min: %<OutMin>
      | %<Description>
  ActionPort : ActionPort  ActionPortLabel=case [ 2 ]:
  IVT_LT1 : Lookup_n-D  NumberOfTableDimensions=1  BreakpointsForDimension1=C02MTLKV.sArrR1  Table=C02MTLKV.sArrT1  ExtrapMethod=Clip  UseLastTableValue=on  InternalRulePriority=Speed
      settings: AttributesFormatString=%<UseLastTableValue>
  sMtrTempLT1_now : Outport
  wires:
  IVT_LT1/1 -> sMtrTempLT1_now/1  "sMtrTempLT1_now"
  sIgbtTemp_R/1 -> IVT_LT1/1

== system c02_SubAdc/Ftn_CalMtrTemp_Tnow/Nftn_MtrTempSensBStp2 ==
  note: Input:
      | Description:
      | Output:
  sIgbtTemp_R : Inport  Description=|  OutMin=0  OutMax=4.9e+05
      | ■ 대표값: 2062
      | ■ 설명: Igbt 온도 센서의 저항값
      settings: AttributesFormatString=|
      | ■ SWC Name: %<Parent>
      | ■ DataType: single
      | ■ Max: %<OutMax>
      | ■ Min: %<OutMin>
      | %<Description>
  ActionPort : ActionPort  ActionPortLabel=case [ 3 ]:
  IVT_LT2 : Lookup_n-D  NumberOfTableDimensions=1  BreakpointsForDimension1=C02MTLKV.sArrR2  Table=C02MTLKV.sArrT2  ExtrapMethod=Clip  UseLastTableValue=on  InternalRulePriority=Speed
      settings: AttributesFormatString=%<UseLastTableValue>
  sMtrTempLT2_now : Outport
  wires:
  sIgbtTemp_R/1 -> IVT_LT2/1
  IVT_LT2/1 -> sMtrTempLT2_now/1  "sMtrTempLT2_now"

== system c02_SubAdc/Ftn_CalMtrTemp_Tnow/Nftn_MtrTempSensBStp3 ==
  note: Input:
      | Description:
      | Output:
  sIgbtTemp_R : Inport  Description=|  OutMin=0  OutMax=4.9e+05
      | ■ 대표값: 2062
      | ■ 설명: Igbt 온도 센서의 저항값
      settings: AttributesFormatString=|
      | ■ SWC Name: %<Parent>
      | ■ DataType: single
      | ■ Max: %<OutMax>
      | ■ Min: %<OutMin>
      | %<Description>
  ActionPort : ActionPort  ActionPortLabel=case [ 4 ]:
  IVT_LT3 : Lookup_n-D  NumberOfTableDimensions=1  BreakpointsForDimension1=C02MTLKV.sArrR3  Table=C02MTLKV.sArrT3  ExtrapMethod=Clip  UseLastTableValue=on  InternalRulePriority=Speed
      settings: AttributesFormatString=%<UseLastTableValue>
  sMtrTempLT3_now : Outport
  wires:
  IVT_LT3/1 -> sMtrTempLT3_now/1  "sMtrTempLT3_now"
  sIgbtTemp_R/1 -> IVT_LT3/1

== system c02_SubAdc/Ftn_CalMtrTemp_Tnow/Nftn_MtrTempSensBStp4 ==
  note: Input:
      | Description:
      | Output:
  sIgbtTemp_R : Inport  Description=|  OutMin=0  OutMax=4.9e+05
      | ■ 대표값: 2062
      | ■ 설명: Igbt 온도 센서의 저항값
  ActionPort : ActionPort  ActionPortLabel=case [ 5 ]:
  IVT_LT4 : Lookup_n-D  NumberOfTableDimensions=1  BreakpointsForDimension1=C02MTLKV.sArrR4  Table=C02MTLKV.sArrT4  ExtrapMethod=Clip  UseLastTableValue=on  InternalRulePriority=Speed
      settings: AttributesFormatString=%<UseLastTableValue>
  sMtrTempLT4_now : Outport
  wires:
  sIgbtTemp_R/1 -> IVT_LT4/1
  IVT_LT4/1 -> sMtrTempLT4_now/1  "sMtrTempLT4_now"

== system c02_SubAdc/Ftn_CalMtrTemp_Tnow/Nftn_MtrTempSensBStp5 ==
  note: Input:
      | Description:
      | Output:
  ActionPort : ActionPort  ActionPortLabel=default:
  CB_sSCaseDflt_now : Constant  Value=0  OutDataTypeStr=single
  sSCaseDflt_now : Outport
  wires:
  CB_sSCaseDflt_now/1 -> sSCaseDflt_now/1  "sSCaseDflt_now"

== stateflow chart c02_SubAdc/Ftn_CalMtrTemp_R/Chart_MtrTempSensR ==
  (default) -> (junction 4)
  (junction 4) -> (junction 59) : {
      | sTempVlt = (sAdcMtrTempSens * sMtrNtcResolut + sMtrNtcHwOffset)*sMtrNtcHwGain;
      | sMtrTemp_R = -sTempVlt * sMtrNtcR0 / (sTempVlt - sMtrNtcV0);
      | }
  data: sAdcMtrTempSens input; sMtrNtcResolut input; sMtrNtcHwOffset input; sMtrNtcHwGain input; sTempVlt local single; sMtrNtcR0 input; sMtrNtcV0 input; sMtrTemp_R output single =570

== stateflow chart c02_SubAdc/Ftn_CalMtrTemp_RIndex1/Chart_IgbtTempSensA ==
  (default) -> (junction 79)
  (junction 79) -> (junction 80) [order 1] : [sMtrTemp_R < sArrDivR1]
  (junction 79) -> (junction 81) [order 2]
  (junction 80) -> (junction 88) : {
      | uMtrTemp_RIndex = C_u16_1;
      | }
  (junction 81) -> (junction 82) [order 1] : [sMtrTemp_R < sArrDivR2]
  (junction 81) -> (junction 83) [order 2]
  (junction 82) -> (junction 87) : {
      | uMtrTemp_RIndex = C_u16_2;
      | }
  (junction 83) -> (junction 84) [order 1] : [sMtrTemp_R < sArrDivR3]
  (junction 83) -> (junction 85) [order 2]
  (junction 84) -> (junction 86) : {
      | uMtrTemp_RIndex = C_u16_3;
      | }
  (junction 85) -> (junction 90) [order 1] : [sMtrTemp_R < sArrDivR4]
  (junction 85) -> (junction 89) [order 2] : {
      | uMtrTemp_RIndex = C_u16_5;
      | }
  (junction 90) -> (junction 92) : {
      | uMtrTemp_RIndex = C_u16_4;
      | }
  (junction 92) -> (junction 89)
  (junction 86) -> (junction 92)
  (junction 87) -> (junction 86)
  (junction 88) -> (junction 87)
  (junction 89) -> (junction 103)
  data: uMtrTemp_RIndex output uint16 =CnstNr.C_u16_1; sMtrTemp_R input; sArrDivR1 input; sArrDivR2 input; sArrDivR3 input; sArrDivR4 input; C_u16_1 input size=[1 1] =1; C_u16_2 input size=[1 1] =2; C_u16_3 input size=[1 1] =3; C_u16_4 input size=[1 1] =4; C_u16_5 input size=[1 1] =5

== stateflow chart c02_SubAdc/Ftn_CalIvtTemp_RIndex/Chart_IgbtTempSensA ==
  (default) -> (junction 79)
  (junction 79) -> (junction 80) [order 1] : [sIvtTemp_R < sArrDivR1]
  (junction 79) -> (junction 81) [order 2]
  (junction 80) -> (junction 88) : {
      | uIvtTemp_RIndex = C_u16_1;
      | }
  (junction 81) -> (junction 82) [order 1] : [sIvtTemp_R < sArrDivR2]
  (junction 81) -> (junction 83) [order 2]
  (junction 82) -> (junction 87) : {
      | uIvtTemp_RIndex = C_u16_2;
      | }
  (junction 83) -> (junction 84) [order 1] : [sIvtTemp_R < sArrDivR3]
  (junction 83) -> (junction 85) [order 2]
  (junction 84) -> (junction 86) : {
      | uIvtTemp_RIndex = C_u16_3;
      | }
  (junction 85) -> (junction 90) [order 1] : [sIvtTemp_R < sArrDivR4]
  (junction 85) -> (junction 89) [order 2] : {
      | uIvtTemp_RIndex = C_u16_5;
      | }
  (junction 90) -> (junction 92) : {
      | uIvtTemp_RIndex = C_u16_4;
      | }
  (junction 92) -> (junction 89)
  (junction 86) -> (junction 92)
  (junction 87) -> (junction 86)
  (junction 88) -> (junction 87)
  (junction 89) -> (junction 103)
  data: uIvtTemp_RIndex output uint16 =CnstNr.C_u16_5; sIvtTemp_R input; sArrDivR1 input; sArrDivR2 input; sArrDivR3 input; sArrDivR4 input; C_u16_1 input size=[1 1] =1; C_u16_2 input size=[1 1] =2; C_u16_3 input size=[1 1] =3; C_u16_4 input size=[1 1] =4; C_u16_5 input size=[1 1] =5

== stateflow chart c02_SubAdc/Ftn_CalIvtTemp_R/Chart_IvtTempSensR ==
  (default) -> (junction 4)
  (junction 4) -> (junction 59) : {
      | sTempVlt = (sAdcIvtTempSens * sIgbtNtcResolut + sIgbtNtcHwOffset)*sIgbtNtcHwGain;
      | sIvtTemp_R = -sTempVlt * sIgbtNtcR0 / (sTempVlt - sIgbtNtcV0);
      | }
  data: sAdcIvtTempSens input; sIgbtNtcResolut input; sIgbtNtcHwOffset input; sIgbtNtcHwGain input; sTempVlt local single; sIgbtNtcR0 input; sIgbtNtcV0 input; sIvtTemp_R output single =25000
